simulink model "DistCtrl_PI"  (R2017a)
settings: Solver=FixedStepDiscrete  StartTime=0.0  StopTime=10  FixedStep=0.01  RelTol=1e-3
PreLoadFcn:
  | robotParameters;
undefined symbols (not defined in the file or in its folder): motorIp, motorSp, ticksPerRot, wheelR
libraries: mobileRoboticsTrainingLib x5, simulink x1
settings Model: Creator=sseshadr  LastModifiedBy=shiremat

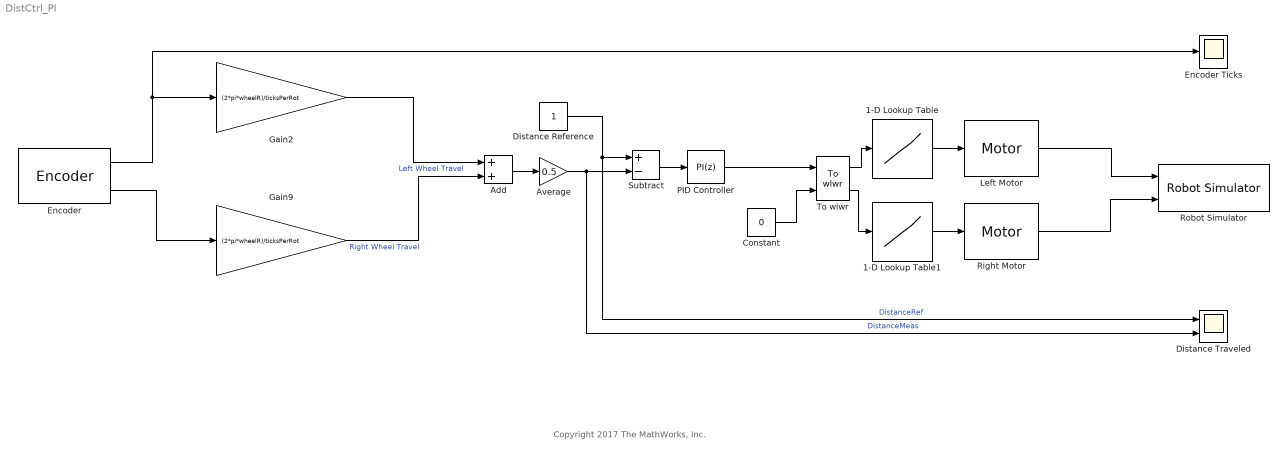
== system DistCtrl_PI ==
  note: Copyright 2017 The MathWorks, Inc.
  1-D Lookup Table : Lookup_n-D  NumberOfTableDimensions=1  BreakpointsForDimension1=motorSp  Table=motorIp  ExtrapMethod=Clip  InternalRulePriority=Speed  RndMeth=Simplest  InputSameDT=on
  1-D Lookup Table1 : Lookup_n-D  NumberOfTableDimensions=1  BreakpointsForDimension1=motorSp  Table=motorIp  ExtrapMethod=Clip  InternalRulePriority=Speed  RndMeth=Simplest  InputSameDT=on
  Add : Sum
  Average : Gain  Gain=0.5
  Constant : Constant  Value=0
  Distance Reference : Constant
  Distance Traveled : Scope  NumInputPorts=2
  Encoder : mobileRoboticsTrainingLib/Encoder  axleLength=axleLength  wheelR=wheelR  ticksPerRot=ticksPerRot
      settings: SourceProductName=Mobile Robotics Training Library
  Encoder Ticks : Scope
  Gain2 : Gain  Gain=(2*pi*wheelR)/ticksPerRot
  Gain9 : Gain  Gain=(2*pi*wheelR)/ticksPerRot
  Left Motor : mobileRoboticsTrainingLib/Motor  motorPlant=wheelMotorModel  sensorType=Speed
      settings: SourceProductName=Mobile Robotics Training Library
  PID Controller : simulink/Continuous/PID Controller  Controller=PI  TimeDomain=Discrete-time  SampleTime=-1  IntegratorMethod=Forward Euler  FilterMethod=Forward Euler  Form=Parallel  UseFilter=off  ControllerParametersSource=internal  P=1.1  I=0.2  D=-0.0140783779685636  N=151.701833251505  InitialConditionSource=internal  InitialConditionForIntegrator=0  InitialConditionForFilter=0  ExternalReset=none  LimitOutput=on  UpperSaturationLimit=0.6  LowerSaturationLimit=-0.6  LinearizeAsGain=on  AntiWindupMode=clamping  Kb=1  TrackingMode=off  Kt=1  PParamMin=[]  PParamMax=[]  IParamMin=[]  IParamMax=[]  DParamMin=[]  DParamMax=[]  NParamMin=[]  NParamMax=[]  KbParamMin=[]  KbParamMax=[]  KtParamMin=[]  KtParamMax=[]  POutMin=[]  POutMax=[]  IOutMin=[]  IOutMax=[]  DOutMin=[]  DOutMax=[]  NOutMin=[]  NOutMax=[]  KbOutMin=[]  KbOutMax=[]  KtOutMin=[]  KtOutMax=[]  IntegratorOutMin=[]  IntegratorOutMax=[]  FilterOutMin=[]  FilterOutMax=[]  SumOutMin=[]  SumOutMax=[]  SumI1OutMin=[]  SumI1OutMax=[]  SumI2OutMin=[]  SumI2OutMax=[]  SumI3OutMin=[]  SumI3OutMax=[]  SumDOutMin=[]  SumDOutMax=[]  SaturationOutMin=[]  SaturationOutMax=[]  IntegratorContinuousStateAttributes=''  IntegratorStateMustResolveToSignalObject=off  IntegratorRTWStateStorageClass=Auto  FilterContinuousStateAttributes=''  FilterStateMustResolveToSignalObject=off  FilterRTWStateStorageClass=Auto  DifferentiatorICPrevScaledInput=0  DifferentiatorOutMin=[]  DifferentiatorOutMax=[]  InitialConditionSetting=Output
  Right Motor : mobileRoboticsTrainingLib/Motor  motorPlant=wheelMotorModel  sensorType=Speed
      settings: SourceProductName=Mobile Robotics Training Library
  Robot Simulator : mobileRoboticsTrainingLib/Robot Simulator  Priority=99  mapVar=[]  startX=2  startY=2  startTheta=0  axleLength=axleLength  wheelR=wheelR
  Subtract : Sum  Inputs=+-
  To wlwr : mobileRoboticsTrainingLib/To wlwr  axleLength=0.1  wheelR=0.05
  wires:
  Average/1 -> Subtract/2, Distance Traveled/2  "DistanceMeas"
  Gain2/1 -> Add/1  "Left Wheel Travel"
  Add/1 -> Average/1
  Gain9/1 -> Add/2  "Right Wheel Travel"
  Encoder/1 -> Gain2/1, Encoder Ticks/1
  Encoder/2 -> Gain9/1
  Constant/1 -> To wlwr/2
  PID Controller/1 -> To wlwr/1
  To wlwr/1 -> 1-D Lookup Table/1
  1-D Lookup Table/1 -> Left Motor/1
  1-D Lookup Table1/1 -> Right Motor/1
  Left Motor/1 -> Robot Simulator/1
  To wlwr/2 -> 1-D Lookup Table1/1
  Right Motor/1 -> Robot Simulator/2
  Distance Reference/1 -> Distance Traveled/1, Subtract/1  "DistanceRef"
  Subtract/1 -> PID Controller/1
